simulink model "Designator_Sim"  (R2025b)
settings: Solver=ode4  StartTime=0.0  StopTime=10.0  RelTol=1e-3
undefined symbols (not defined in the file): d_divergence, d_efficiency, d_h_error, d_pulse_duration, d_pulse_energy, d_pulse_frequency, d_raycount, d_v_error
settings Model: DataDictionary=Designator_Sim_data.sldd  Creator=mauro  LastModifiedBy=mauro

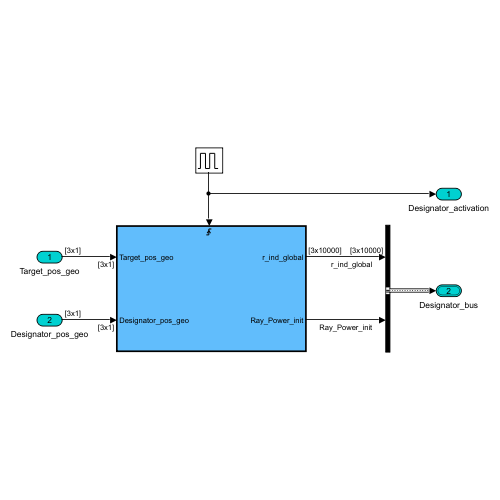
[thumbnail: Simulink's stored preview of the top-level diagram]
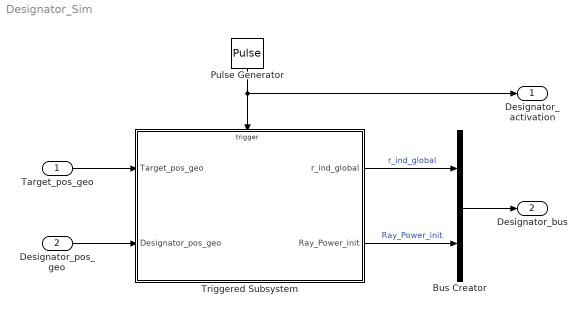
== system Designator_Sim ==
  Target_pos_geo : Inport  PortDimensions=[3 1]
  Designator_pos_geo : Inport  Port=2  PortDimensions=[3 1]
  Bus Creator : BusCreator  Inputs=2  OutDataTypeStr=Bus: Designator_bus  NonVirtualBus=on
  Pulse Generator : DiscretePulseGenerator  PulseType=Time based  Period=1/d_pulse_frequency  PulseWidth=d_pulse_frequency  PhaseDelay=0.01
  Triggered Subsystem : Subsystem  TreatAsAtomicUnit=on
  Designator_activation : Outport
  Designator_bus : Outport  Port=2  OutDataTypeStr=Bus: Designator_bus  BusOutputAsStruct=on
  wires:
  Pulse Generator/1 -> Designator_activation/1, Triggered Subsystem/Trigger
  Triggered Subsystem/1(r_ind_global) -> Bus Creator/1  "r_ind_global"
  Triggered Subsystem/2(Ray_Power_init) -> Bus Creator/2  "Ray_Power_init"
  Bus Creator/1 -> Designator_bus/1
  Designator_pos_geo/1 -> Triggered Subsystem/2(Designator_pos_geo)
  Target_pos_geo/1 -> Triggered Subsystem/1(Target_pos_geo)

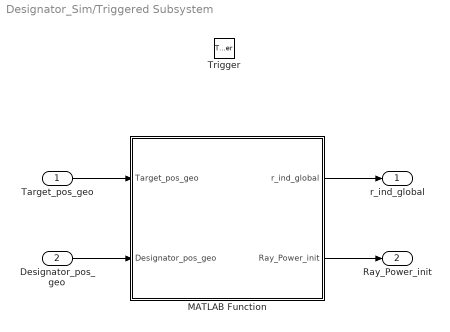
== system Designator_Sim/Triggered Subsystem ==
  Target_pos_geo : Inport
  Designator_pos_geo : Inport  Port=2
  Trigger : TriggerPort  VariantControl=(inherit)  PortDimensions=1
  MATLAB Function : MATLAB Function  TreatAsAtomicUnit=on
  r_ind_global : Outport
  Ray_Power_init : Outport  Port=2
  wires:
  MATLAB Function/1(r_ind_global) -> r_ind_global/1
  MATLAB Function/2(Ray_Power_init) -> Ray_Power_init/1
  Designator_pos_geo/1 -> MATLAB Function/2(Designator_pos_geo)
  Target_pos_geo/1 -> MATLAB Function/1(Target_pos_geo)

== matlab function Designator_Sim/Triggered Subsystem/MATLAB Function ==
  data: Target_pos_geo input; Designator_pos_geo input; d_h_error parameter; r_ind_global output; Ray_Power_init output; d_efficiency parameter; d_pulse_duration parameter; d_pulse_energy parameter; d_divergence parameter; d_raycount parameter; d_v_error parameter
function [r_ind_global, Ray_Power_init] = Ray_pulse_generator(Target_pos_geo,Designator_pos_geo,d_h_error,d_efficiency, d_pulse_duration, d_pulse_energy, d_divergence, d_raycount, d_v_error)

X_axis_designator       = (Target_pos_geo-Designator_pos_geo)/norm(Target_pos_geo-Designator_pos_geo);
Rot_matrix_designator   = [X_axis_designator(1), -(1/sqrt(1-X_axis_designator(3)^2))*X_axis_designator(2), -(1/sqrt(1-X_axis_designator(3)^2))*X_axis_designator(1)*X_axis_designator(3);
                           X_axis_designator(2), 1/sqrt(1-X_axis_designator(3)^2)*X_axis_designator(1), -(1/sqrt(1-X_axis_designator(3)^2))*X_axis_designator(2)*X_axis_designator(3);
                           X_axis_designator(3), 0, 1/(1/sqrt(1-X_axis_designator(3)^2))];

    
d_aim           = [1;tan(d_h_error*randn());tan(d_v_error*randn())];
r_ind           = ones(d_raycount,1)*d_aim'+ [zeros(d_raycount,1),tan(d_divergence/2)*randn(d_raycount,1),tan(d_divergence/2)*randn(d_raycount,1)];
r_ind           = r_ind';% Size = [3,d_raycount]
norms = sqrt(sum(r_ind.^2, 1)); 
r_ind = r_ind ./ norms; 
r_ind_global = Rot_matrix_designator * r_ind;

Ray_Power_init  = d_pulse_energy/d_pulse_duration*d_efficiency/d_raycount;

end
